simulink model "Lin"  (Simulink 7.2)
settings: Solver=ode45  StartTime=0.0  StopTime=0.5  RelTol=1e-3
libraries: simulink x1
settings Model: Creator=Admin  LastModifiedBy=Admin
settings OptimizationCC: InitFltsAndDblsToZero=on
settings DebuggingCC: SaveWithParameterizedLinksMsg=none  SignalResolutionControl=TryResolveAllWithWarning  MultiTaskDSMMsg=warning  MultiTaskCondExecSysMsg=none  StrictBusMsg=None
settings RTWCC: IncludeERTFirstTime=on
settings GRTTargetCC: TargetFcnLib=ansi_tfl_tmw.mat

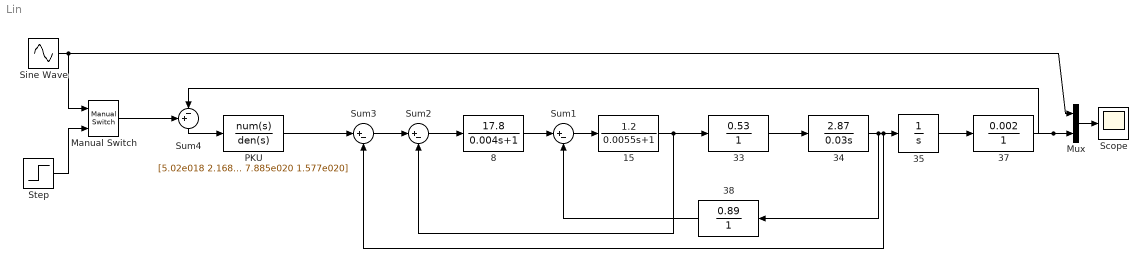
== system Lin ==
  15 : TransferFcn  Numerator=[1.2]  Denominator=[0.0055 1]
  33 : TransferFcn  Numerator=[0.53]  Denominator=[1]
  34 : TransferFcn  Numerator=[2.87]  Denominator=[0.03 0]
  35 : TransferFcn  Denominator=[1 0]
  37 : TransferFcn  Numerator=[0.002]  Denominator=[1]
  38 : TransferFcn  Orientation=left  Numerator=[0.89]  Denominator=[1]
  8 : TransferFcn  Numerator=[17.8]  Denominator=[0.004 1]
  Manual Switch : simulink/Signal Routing/Manual Switch  SystemSampleTime=-1  sw=1  action=0  varsize=off
  Mux : Mux  Inputs=2
  PKU : TransferFcn  Numerator=[5.02e018 2.168e021 5.151e024 2.595e026 0]  Denominator=[0.09884 1.84e004 1.079e009 2.509e013 2.393e017 7.885e020 1.577e020]
  Scope : Scope
      settings: YMin=0  YMax=1
  Sine Wave : Sin  Frequency=500  SampleTime=0
  Step : Step  Time=0  SampleTime=0
  Sum1 : Sum  Inputs=|+-  OutDataType=sfix(16)  OutScaling=2^0
  Sum2 : Sum  Inputs=|+-  OutDataType=sfix(16)  OutScaling=2^0
  Sum3 : Sum  Inputs=|+-  OutDataType=sfix(16)  OutScaling=2^0
  Sum4 : Sum  Orientation=down  Inputs=+-|  OutDataType=sfix(16)  OutScaling=2^0
  wires:
  34/1 -> 38/1, 35/1, Sum3/2
  38/1 -> Sum1/2
  8/1 -> Sum1/1
  Sum3/1 -> Sum2/1
  Sum2/1 -> 8/1
  Sum4/1 -> PKU/1
  37/1 -> Sum4/2, Mux/2
  Mux/1 -> Scope/1
  Manual Switch/1 -> Sum4/1
  Sine Wave/1 -> Manual Switch/1, Mux/1
  Step/1 -> Manual Switch/2
  Sum1/1 -> 15/1
  15/1 -> 33/1, Sum2/2
  33/1 -> 34/1
  35/1 -> 37/1
  PKU/1 -> Sum3/1
